simulink model "sampleModel1740"  (R2023a)
settings: Solver=VariableStepAuto  StartTime=0.0  StopTime=10.0  RelTol=1e-3
libraries: hdlsllib x5
settings Model: Creator=user1  LastModifiedBy=user1

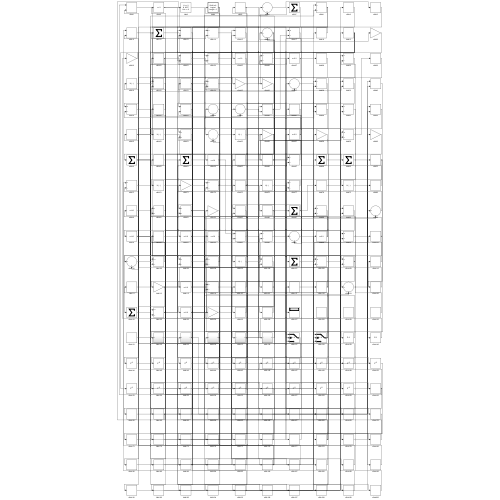
[thumbnail: Simulink's stored preview of the top-level diagram]
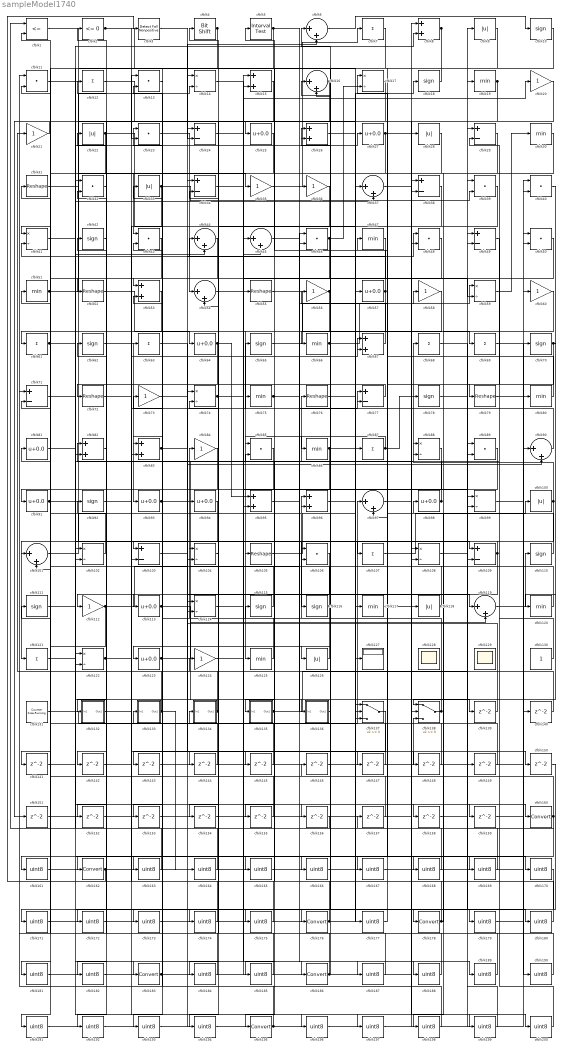
== system sampleModel1740 ==
  cfblk1 : RelationalOperator  Operator=<=  OutDataTypeStr=boolean  InputSameDT=off
  cfblk{10,18,42,62,65,70,78,92,110..111,115..116} (12 alike) : Signum
  cfblk{9,22,28,33,100,118,126} (7 alike) : Abs  SaturateOnIntegerOverflow=off
  cfblk{6,16,37,44..45,54,90,97,101,119} (10 alike) : Sum  Inputs=|++
  cfblk{14,17,41,59,74,88,99,102,104,108,114,122} (12 alike) : Product  Inputs=*/  RndMeth=Zero  SaturateOnIntegerOverflow=on
  cfblk{24,29,34,38,49,71,77,103,109} (9 alike) : Sum  Inputs=+-
  cfblk{31,52,55,72,76,79,105} (7 alike) : Reshape
  cfblk{11,13,23,32,39..40,43,46,48,50,85,89,106} (13 alike) : DotProduct  OutDataTypeStr=Inherit: Inherit via internal rule
  cfblk{7,12,61,63,68..69,87,107,121} (9 alike) : Sum  Inputs=+
  cfblk{20..21,35..36,56,58,60,73,84,112,124} (11 alike) : Gain
  cfblk{25,27,57,64,81,91,93..94,98,113,123} (11 alike) : Bias  Bias=0.0  SaturateOnIntegerOverflow=off
  cfblk{19,30,47,51,66,75,80,86,117,120,125} (11 alike) : MinMax
  cfblk127 : Display
  cfblk128 : Scope
      settings: Floating=on
  cfblk129 : Scope
      settings: Floating=on
  cfblk130 : Constant  SampleTime=-1
  cfblk131 : hdlsllib/Sources/Counter Free-Running  NumBits=16  tsamp=-1
  cfblk132 : Subsystem
      settings: LibrarySourceBlock=|
      | hdlsllib/Ports &
      | Subsystems/Subsystem
  cfblk133 : Subsystem
      settings: LibrarySourceBlock=|
      | hdlsllib/Ports &
      | Subsystems/Subsystem
  cfblk134 : Subsystem
      settings: LibrarySourceBlock=|
      | hdlsllib/Ports &
      | Subsystems/Subsystem
  cfblk135 : Subsystem
      settings: LibrarySourceBlock=|
      | hdlsllib/Ports &
      | Subsystems/Subsystem
  cfblk136 : Subsystem
      settings: LibrarySourceBlock=|
      | hdlsllib/Ports &
      | Subsystems/Subsystem
  cfblk137 : Switch  SaturateOnIntegerOverflow=off  InputSameDT=off
  cfblk138 : Switch  SaturateOnIntegerOverflow=off  InputSameDT=off
  cfblk{139..159} (21 alike) : Delay  SampleTime=1
  cfblk{8,15,26,53,67,82..83,95..96} (9 alike) : Sum
  cfblk{160,162,176,178,183,186,195} (7 alike) : DataTypeConversion  SaturateOnIntegerOverflow=off  RndMeth=Floor
  cfblk{161,163..175,177,179..182,184..185,187..194,196..200} (34 alike) : DataTypeConversion  OutDataTypeStr=uint8  SaturateOnIntegerOverflow=off  RndMeth=Floor
  cfblk2 : hdlsllib/Logic and Bit Operations/Compare To Zero  relop=<=  OutDataTypeStr=boolean
  cfblk3 : hdlsllib/Logic and Bit Operations/Detect Fall Nonpositive  vinit=0  OutDataTypeStr=boolean
  cfblk4 : hdlsllib/Logic and Bit Operations/Bit Shift  mode=Shift Left Logical  N=0
  cfblk5 : hdlsllib/Logic and Bit Operations/Interval Test  IntervalClosedRight=on  uplimit=0.5  IntervalClosedLeft=on  lowlimit=-0.5  OutDataTypeStr=boolean
  wires:
  cfblk116/1 -> cfblk73/1, cfblk184/1
  cfblk18/1 -> cfblk103/1
  cfblk57/1 -> cfblk125/1, cfblk5/1, cfblk41/2
  cfblk47/1 -> cfblk176/1
  cfblk133/1(Out1) -> cfblk21/1, cfblk164/1
  cfblk23/1 -> cfblk54/1
  cfblk115/1 -> cfblk81/1
  cfblk94/1 -> cfblk121/1
  cfblk131/1 -> cfblk97/1
  cfblk52/1 -> cfblk64/1
  cfblk20/1 -> cfblk105/1
  cfblk130/1 -> cfblk82/1
  cfblk101/1 -> cfblk96/1
  cfblk35/1 -> cfblk7/1
  cfblk77/1 -> cfblk72/1
  cfblk118/1 -> cfblk84/1, cfblk77/1
  cfblk59/1 -> cfblk30/1
  cfblk62/1 -> cfblk93/1
  cfblk99/1 -> cfblk40/1
  cfblk123/1 -> cfblk76/1, cfblk119/2, cfblk67/1
  cfblk119/1 -> cfblk110/1
  cfblk10/1 -> cfblk97/2
  cfblk126/1 -> cfblk123/1
  cfblk55/1 -> cfblk69/1
  cfblk16/1 -> cfblk41/1, cfblk152/1
  cfblk110/1 -> cfblk56/1
  cfblk117/1 -> cfblk160/1
  cfblk31/1 -> cfblk35/1
  cfblk78/1 -> cfblk39/1
  cfblk100/1 -> cfblk101/1, cfblk88/1
  cfblk40/1 -> cfblk138/1
  cfblk80/1 -> cfblk17/1
  cfblk86/1 -> cfblk95/2, cfblk158/1
  cfblk44/1 -> cfblk53/1
  cfblk96/1 -> cfblk18/1
  cfblk125/1 -> cfblk104/1
  cfblk28/1 -> cfblk43/1
  cfblk22/1 -> cfblk137/1, cfblk91/1
  cfblk38/1 -> cfblk195/1
  cfblk7/1 -> cfblk61/1
  cfblk138/1 -> cfblk96/2, cfblk33/1
  cfblk14/1 -> cfblk55/1
  cfblk32/1 -> cfblk162/1
  cfblk98/1 -> cfblk68/1, cfblk26/2
  cfblk90/1 -> cfblk65/1
  cfblk102/1 -> cfblk51/1
  cfblk136/1(Out1) -> cfblk26/1
  cfblk27/1 -> cfblk28/1, cfblk46/2
  cfblk93/1 -> cfblk113/1, cfblk147/1
  cfblk49/1 -> cfblk79/1
  cfblk113/1 -> cfblk46/1, cfblk137/3
  cfblk107/1 -> cfblk100/1
  cfblk37/1 -> cfblk118/1
  cfblk134/1(Out1) -> cfblk23/1, cfblk194/1
  cfblk51/1 -> cfblk14/2, cfblk37/2
  cfblk75/1 -> cfblk59/1, cfblk188/1
  cfblk65/1 -> cfblk9/1
  cfblk71/1 -> cfblk183/1
  cfblk19/1 -> cfblk86/1, cfblk66/1, cfblk48/2, cfblk163/1, cfblk193/1
  cfblk34/1 -> cfblk186/1
  cfblk82/1 -> cfblk42/1
  cfblk70/1 -> cfblk120/1, cfblk167/1
  cfblk8/1 -> cfblk126/1, cfblk153/1
  cfblk60/1 -> cfblk178/1
  cfblk6/1 -> cfblk10/1
  cfblk105/1 -> cfblk37/1
  cfblk58/1 -> cfblk103/2
  cfblk39/1 -> cfblk107/1
  cfblk61/1 -> cfblk136/1(In1), cfblk44/2, cfblk156/1
  cfblk4/1 -> cfblk102/2, cfblk23/2
  cfblk11/1 -> cfblk25/1
  cfblk109/1 -> cfblk112/1, cfblk106/1
  cfblk91/1 -> cfblk116/1, cfblk109/2, cfblk88/2
  cfblk103/1 -> cfblk6/2
  cfblk104/1 -> cfblk74/2
  cfblk33/1 -> cfblk39/2, cfblk83/2
  cfblk66/1 -> cfblk58/1, cfblk16/2, cfblk169/1
  cfblk111/1 -> cfblk8/2
  cfblk54/1 -> cfblk99/2
  cfblk15/1 -> cfblk82/2
  cfblk122/1 -> cfblk63/1, cfblk75/1
  cfblk135/1(Out1) -> cfblk49/2, cfblk77/2
  cfblk12/1 -> cfblk127/1
  cfblk64/1 -> cfblk95/1, cfblk142/1
  cfblk81/1 -> cfblk27/1
  cfblk25/1 -> cfblk122/2
  cfblk120/1 -> cfblk92/1
  cfblk95/1 -> cfblk137/2
  cfblk74/1 -> cfblk4/1, cfblk20/1
  cfblk30/1 -> cfblk135/1(In1)
  cfblk84/1 -> cfblk101/2
  cfblk87/1 -> cfblk85/1, cfblk78/1
  cfblk2/1 -> cfblk36/1, cfblk24/2
  cfblk46/1 -> cfblk52/1, cfblk17/2
  cfblk3/1 -> cfblk24/1
  cfblk67/1 -> cfblk16/1
  cfblk42/1 -> cfblk12/1
  cfblk24/1 -> cfblk59/2
  cfblk5/1 -> cfblk109/1, cfblk83/1
  cfblk83/1 -> cfblk119/1, cfblk90/2
  cfblk112/1 -> cfblk94/1, cfblk67/2, cfblk161/1
  cfblk1/1 -> cfblk87/1
  cfblk56/1 -> cfblk132/1(In1), cfblk182/1
  cfblk73/1 -> cfblk48/1
  cfblk63/1 -> cfblk139/1
  cfblk139/1 -> cfblk14/1
  cfblk79/1 -> cfblk140/1
  cfblk140/1 -> cfblk102/1
  cfblk43/1 -> cfblk141/1
  cfblk137/1 -> cfblk143/1
  cfblk143/1 -> cfblk138/3
  cfblk17/1 -> cfblk144/1
  cfblk144/1 -> cfblk74/1
  cfblk9/1 -> cfblk145/1
  cfblk145/1 -> cfblk11/2
  cfblk146/1 -> cfblk40/2
  cfblk147/1 -> cfblk6/1
  cfblk132/1(Out1) -> cfblk148/1
  cfblk148/1 -> cfblk1/2
  cfblk68/1 -> cfblk149/1
  cfblk149/1 -> cfblk122/1
  cfblk26/1 -> cfblk150/1
  cfblk21/1 -> cfblk151/1
  cfblk151/1 -> cfblk8/1
  cfblk153/1 -> cfblk104/2
  cfblk36/1 -> cfblk154/1
  cfblk154/1 -> cfblk138/2
  cfblk88/1 -> cfblk155/1
  cfblk155/1 -> cfblk54/2
  cfblk156/1 -> cfblk1/1
  cfblk157/1 -> cfblk85/2
  cfblk158/1 -> cfblk19/1
  cfblk92/1 -> cfblk159/1
  cfblk159/1 -> cfblk70/1
  cfblk160/1 -> cfblk157/1, cfblk31/1, cfblk191/1
  cfblk161/1 -> cfblk117/1
  cfblk162/1 -> cfblk3/1, cfblk80/1
  cfblk163/1 -> cfblk32/1
  cfblk164/1 -> cfblk32/2
  cfblk50/1 -> cfblk165/1
  cfblk165/1 -> cfblk99/1
  cfblk121/1 -> cfblk166/1
  cfblk166/1 -> cfblk50/1
  cfblk167/1 -> cfblk50/2
  cfblk124/1 -> cfblk168/1
  cfblk168/1 -> cfblk22/1
  cfblk169/1 -> cfblk124/1
  cfblk45/1 -> cfblk170/1
  cfblk150/1 -> cfblk171/1
  cfblk171/1 -> cfblk45/1
  cfblk85/1 -> cfblk172/1
  cfblk172/1 -> cfblk45/2
  cfblk13/1 -> cfblk173/1
  cfblk173/1 -> cfblk57/1
  cfblk170/1 -> cfblk174/1
  cfblk174/1 -> cfblk13/1
  cfblk48/1 -> cfblk175/1
  cfblk175/1 -> cfblk13/2
  cfblk176/1 -> cfblk44/1, cfblk62/1
  cfblk76/1 -> cfblk177/1
  cfblk177/1 -> cfblk47/1
  cfblk178/1 -> cfblk106/2, cfblk15/1, cfblk98/1
  cfblk41/1 -> cfblk179/1
  cfblk179/1 -> cfblk60/1
  cfblk108/1 -> cfblk180/1
  cfblk180/1 -> cfblk115/1
  cfblk53/1 -> cfblk181/1
  cfblk181/1 -> cfblk108/1
  cfblk182/1 -> cfblk108/2
  cfblk183/1 -> cfblk15/2, cfblk43/2, cfblk133/1(In1)
  cfblk184/1 -> cfblk71/1
  cfblk106/1 -> cfblk185/1
  cfblk185/1 -> cfblk71/2
  cfblk186/1 -> cfblk146/1, cfblk2/1, cfblk111/1
  cfblk152/1 -> cfblk187/1
  cfblk187/1 -> cfblk34/1
  cfblk188/1 -> cfblk34/2
  cfblk114/1 -> cfblk189/1
  cfblk189/1 -> cfblk134/1(In1)
  cfblk69/1 -> cfblk190/1
  cfblk190/1 -> cfblk114/1
  cfblk191/1 -> cfblk114/2
  cfblk89/1 -> cfblk192/1
  cfblk192/1 -> cfblk49/1
  cfblk193/1 -> cfblk89/1
  cfblk194/1 -> cfblk89/2
  cfblk195/1 -> cfblk90/1, cfblk53/2
  cfblk72/1 -> cfblk196/1
  cfblk196/1 -> cfblk38/1
  cfblk141/1 -> cfblk197/1
  cfblk197/1 -> cfblk38/2
  cfblk29/1 -> cfblk198/1
  cfblk198/1 -> cfblk11/1
  cfblk97/1 -> cfblk199/1
  cfblk199/1 -> cfblk29/1
  cfblk142/1 -> cfblk200/1
  cfblk200/1 -> cfblk29/2

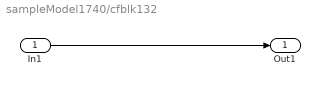
== system sampleModel1740/cfblk132 ==
  In1 : Inport
  Out1 : Outport
  wires:
  In1/1 -> Out1/1

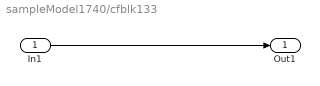
== system sampleModel1740/cfblk133 ==
  In1 : Inport
  Out1 : Outport
  wires:
  In1/1 -> Out1/1

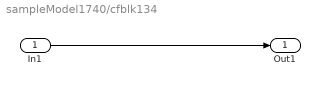
== system sampleModel1740/cfblk134 ==
  In1 : Inport
  Out1 : Outport
  wires:
  In1/1 -> Out1/1

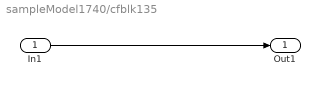
== system sampleModel1740/cfblk135 ==
  In1 : Inport
  Out1 : Outport
  wires:
  In1/1 -> Out1/1

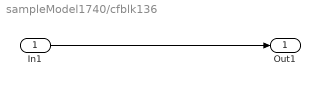
== system sampleModel1740/cfblk136 ==
  In1 : Inport
  Out1 : Outport
  wires:
  In1/1 -> Out1/1
